simulink model "FullModel"  (R2024b)
settings: Solver=ode4  StartTime=0.0  StopTime=60  FixedStep=1e-5  RelTol=1e-3
InitFcn:
  | % Define Simulink sampling time
  | params.Tsam = 1e-5;
  | % Load frequency
  | params.f0=50;
  | %% LCL - filter design
  | % DC link voltage
  | params.Vdc=800;
  | %Switching frequency
  | params.fs=10e3;
  | params.Ts=1/params.fs;
  | params.Filter.Ls_1=1e-3;
  | params.Filter.Ls_2=0.5e-3;
  | params.Filter.Cs = 50e-6;
  | %% PI current-----------
  | params.Tresc=1e-3;
  | params.e=1;
  | params.omega=2*pi/params.Tresc;
  | params.k=1/params.Filter.Ls_1;
  | params.Kpc=2*params.e*params.omega/params.k;
  | params.Kic=params.omega^2/params.k;
  | 
  | %% PI voltage controller-----------
  | params.Tresv=10e-3;
  | params.ev=1;
  | params.omegav=2*pi/params.Tresv;
  | params.kv=1/params.Filter.Cs;
  | params.Kpv=2*params.ev*params.omegav/params.kv;
  | params.Kiv=params.omegav^2/params.kv;
  | params.Pref = 4.5e3;         % 0.5 MW
  | params.Qref = 1000;         % 0.1 Mvar
  | params.Vn   = 110;  % 22 kV line-to-line  →  phase (RMS)
  | params.wn = 2*pi*50;
  | params.Vj = 110;
  | params.XR = 1;
  | 
  | % Đặc tả cực đặt cho pole-placement
  | zeta      = 1;
  | T_setl    = 1;
  | omega_n   = 4/(zeta*T_setl);
  | p1        = -zeta*omega_n + 1i*omega_n*sqrt(1-zeta^2);
  | poles     = [p1, conj(p1), -80, -90, -100];
  | % Controller gain K
  | % K = place(A, B, p);
  | K_now = -[339.437515294446	-37.1962550049616	-155.433559437714	37.2641713114898	3289.76434330323;
  | 287.980448278270	35.5843781184771	-282.198010268474	58.4116660247888	-4058.33626972146];
  | % 3a) Conventional P-loop (fixed gains from your design)
  | Kp = 0.006383815167581;
  | Dp = 2.506338228783948e3;
  | 
  | % 3b) Conventional Q-loop (fixed gains)
  | Kq = 0.076670166944346;
  | Dq = 1.033099625954584;
undefined symbols (not defined in the file or in its folder): Filter, IP, Ls, UDP
libraries: spsSeriesRLCBranchLib x47, spsIdealSwitchLib x26, spsCurrentMeasurementLib x6, spsIGBTDiodeLib x6, rtlab x5, simulink x4, spsVoltageMeasurementLib x4, spsMeanLib x2, spsDCVoltageSourceLib x1, spsThreePhaseSourceLib x1, spsThreePhaseVIMeasurementLib x1, rtio_generic_ip x1
settings Model: Creator=Admin  LastModifiedBy=ACER
settings DataIOCC: SaveOutput=off  DSMLogging=off  SaveTime=off  ReturnWorkspaceOutputs=off
settings OptimizationCC: EfficientMapNaN2IntZero=off  AccelVerboseBuild=on
settings DebuggingCC: UnconnectedInputMsg=warning  UnconnectedOutputMsg=warning  UnconnectedLineMsg=warning
settings HardwareCC: TargetBitPerPointer=64  TargetBitPerSizeT=64  TargetBitPerPtrDiffT=64  TargetLongLongMode=on  TargetIntDivRoundTo=Zero  TargetEndianess=LittleEndian  TargetWordSize=64  TargetHWDeviceType=MATLAB Host  ProdEqTarget=off
settings ModelReferenceCC: EnableRefExpFcnMdlSchedulingChecks=on
settings SFSimCC: CustomCodeUndefinedFunction=UseInterfaceOnly
settings RTWCC: GenerateReport=on  GPUComputeCapability=3.5
settings CodeAppCC: MaxIdLength=128
settings GRTTargetCC: TargetLangStandard=C89/C90 (ANSI)  CombineOutputUpdateFcns=off  GRTInterface=on

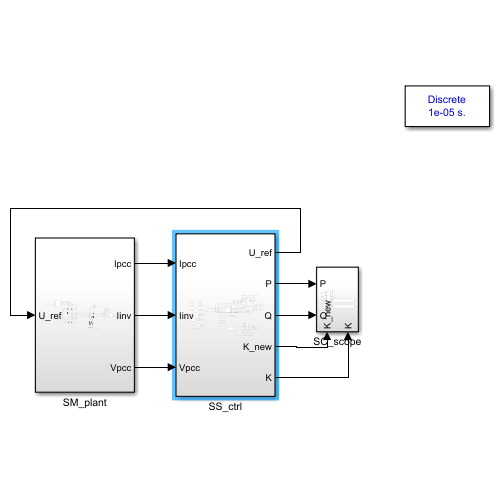
[thumbnail: Simulink's stored preview of the top-level diagram]
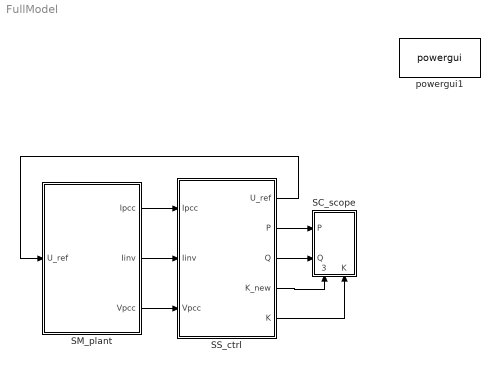
== system FullModel ==
  SC_scope : Subsystem
      settings: PortSchema="{\"entries\":[{\"content\":{\"sides\":[{\"content\":{\"connectorIds\":[\"In1\",\"In2\"]},\"type\":\"ConnectorPlacement.EquallySpacedRectSide\",\"uuid\":\"1d0fbc94-f50e-4dac-aa38-f6c6c0d58e24\"},{\"content\":{\"side\":\"RIGHT\"},\"type\":\"ConnectorPlacement.EquallySpacedRectSide\",\"uuid\":\"cb070a2d-4924-49b4-8117-60b0e85ee68e\"},{\"content\":{\"side\":\"TOP\"},\"type\":\"ConnectorPlacement.EquallySpacedRectSide\",\"uuid\":\"37bb5879-11cc-4540-93be-6819b671c3f0\"},{\"content\":{\"connectorIds\":[\"In3\",\"In4\"],\"side\":\"BOTTOM\"},\"type\":\"ConnectorPlacement.EquallySpacedRectSide\",\"uuid\":\"e4b3a2c0-2caf-4b94-9e11-126344d60f0a\"}]},\"type\":\"ConnectorPlacement.EquallySpacedConnector\",\"uuid\":\"b55f8133-fa8d-4679-9685-8775147a1bfa\"}],\"packageUris\":[\"http://schema.mathworks.com/mf0/Connector/R2020b\"],\"version\":\"1.0\"}"
  SM_plant : Subsystem
  SS_ctrl : Subsystem
  powergui1 : spspowerguiLib/powergui  Priority=1  SimulationMode=Discrete  SampleTime=1e-5  frequency=60  Iterations=50  frequencyindice=0  Pbase=100e6  ErrMax=1e-4  UnitsV=kV  UnitsW=MW  buscounter=0  FunctionMessages=off  echomessages=off  EnableUseOfTLC=off  CurrentSourceSwitches=off  DisableSnubberDevices=off  DisableRonSwitches=off  DisableVfSwitches=off  DisplayEquations=off  AutomaticDiscreteSolvers=on  SolverType=Tustin/Backward Euler (TBE)  Interpol=off  ExternalGateDelay=off  methode=off  Ts=100  x0status=blocks  SPID=on  SwTol=0  HookPort=off  NonlinearTolerance=0  nMaxIteration=15  ContinueOnMaxIteration=off  RestoreLinks=warning  ResistiveCurrentMeasurement=off  Frange=[0:2:500]  Ylog=off  Xlog=on  ShowGrid=off  save=off  variable=ZData  structure=0  ZoomFFT=off  StartTime=0.0  cycles=1  DisplayStyle=1  fundamental=60  FreqAxis=off  MaxFrequency=1000  frequencyindicesteady=1  RmsSteady=1  display=off
  wires:
  SM_plant/1(Ipcc) -> SS_ctrl/1(Ipcc)
  SM_plant/2(Iinv) -> SS_ctrl/2(Iinv)
  SM_plant/3(Vpcc) -> SS_ctrl/3(Vpcc)
  SS_ctrl/1(U_ref) -> SM_plant/1(U_ref)
  SS_ctrl/2(P) -> SC_scope/1(P)
  SS_ctrl/3(Q) -> SC_scope/2(Q)
  SS_ctrl/4(K_new) -> SC_scope/3(K_new)
  SS_ctrl/5(K) -> SC_scope/4(K)

== system FullModel/SC_scope ==
  P : Inport
  Q : Inport  Port=2
  K_new : Inport  Port=3
  K : Inport  Port=4
  Display : Display
  Display1 : Display
  OpComm : rtlab/OpComm  nbport=4  groupe_acq=1  subsys_rate=2e-4  st=0  Synchronization=on  Interpolation=on  Threshold=1.0  Missed_Data=off  Sim_Time=off  Samples=off  dynSigOut=off  from_console=0  warning_done=off  writeOpCommFile=off  Offset=off
      settings: SourceProductName=RT-LAB
  Scope : Scope  NumInputPorts=2
  wires:
  Q/1 -> OpComm/2
  P/1 -> OpComm/1
  OpComm/2 -> Scope/2
  OpComm/1 -> Scope/1
  K_new/1 -> OpComm/3
  OpComm/3 -> Display/1
  K/1 -> OpComm/4
  OpComm/4 -> Display1/1

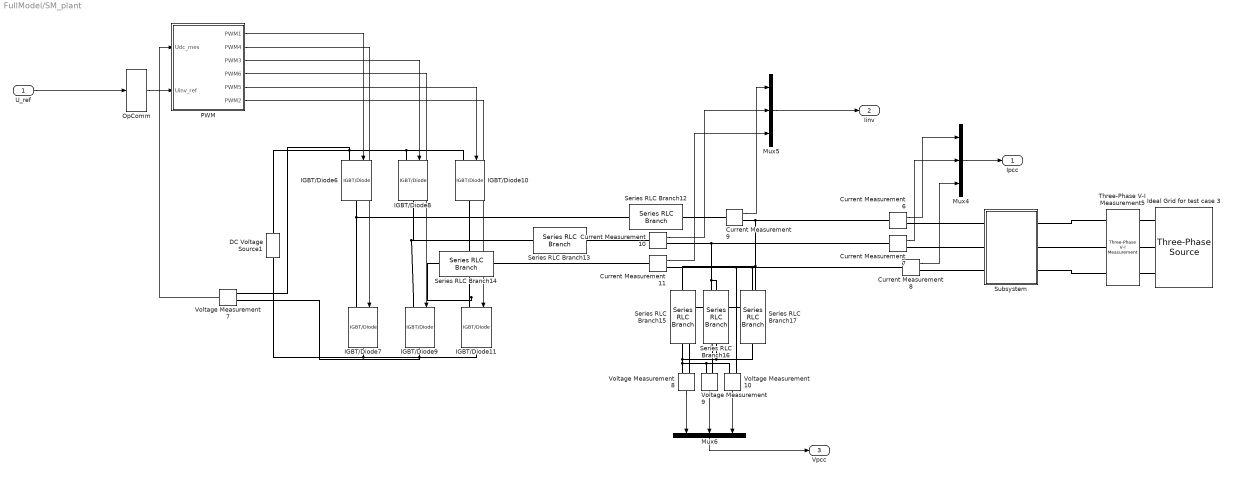
== system FullModel/SM_plant ==
  U_ref : Inport
  Current Measurement{6..11} (6 alike) : spsCurrentMeasurementLib/Current Measurement  PhasorSimulation=off  OutputType=Complex  PSBequivalent=0
  DC Voltage Source1 : spsDCVoltageSourceLib/DC Voltage Source  Amplitude=params.Vdc  Measurements=None
  IGBT/Diode{6..11} (6 alike) : spsIGBTDiodeLib/IGBT//Diode  Ron=1e-3  Rs=1e5  Cs=inf  Measurements=off
  Ideal Grid for test case 3 : spsThreePhaseSourceLib/Three-Phase Source  InternalConnection=Yg  VoltagePhases=off  Voltage=params.Vj*sqrt(3)  PhaseAngle=0  Voltage_phases=[25e3 25e3 25e3]/sqrt(3)  PhaseAngles_phases=[0 -120 +120]  Frequency=params.f0  NonIdealSource=off  SpecifyImpedance=on  Resistance=0.8929  Inductance=16.58e-3  ShortCircuitLevel=params.SCR*params.S_rated  BaseVoltage=params.Vll_rms  XRratio=params.XR  BusType=swing  Pref=1e3  Qref=0  Prefabc=[10e3, 10e3, 10e3]  Qrefabc=[0, 0, 0]  Qmin=-inf  Qmax=inf
  Mux4 : Mux  Inputs=3
  Mux5 : Mux  Inputs=3
  Mux6 : Mux  Inputs=3
  OpComm : rtlab/OpComm  nbport=1  groupe_acq=1  subsys_rate=0  st=0  Synchronization=on  Interpolation=on  Threshold=1.0  Missed_Data=off  Sim_Time=off  Samples=off  dynSigOut=off  from_console=0  warning_done=off  writeOpCommFile=off  Offset=off
      settings: SourceProductName=RT-LAB
  PWM : Subsystem
  Series RLC Branch12 : spsSeriesRLCBranchLib/Series RLC Branch  LConnTagsString=__new0  RConnTagsString=__new0  BranchType=L  Resistance=Filter.Rs_1  Inductance=params.Filter.Ls_1  SetiL0=off  InitialCurrent=1  Capacitance=1e-6  Setx0=off  InitialVoltage=0  Measurements=None
  Series RLC Branch13 : spsSeriesRLCBranchLib/Series RLC Branch  LConnTagsString=__new0  RConnTagsString=__new0  BranchType=L  Resistance=Filter.Rs_1  Inductance=params.Filter.Ls_1  SetiL0=off  InitialCurrent=1  Capacitance=1e-6  Setx0=off  InitialVoltage=0  Measurements=None
  Series RLC Branch14 : spsSeriesRLCBranchLib/Series RLC Branch  LConnTagsString=__new0  RConnTagsString=__new0  BranchType=L  Resistance=Filter.Rs_1  Inductance=params.Filter.Ls_1  SetiL0=off  InitialCurrent=1  Capacitance=1e-6  Setx0=off  InitialVoltage=0  Measurements=None
  Series RLC Branch15 : spsSeriesRLCBranchLib/Series RLC Branch  LConnTagsString=__new0  RConnTagsString=__new0  BranchType=C  Resistance=1  Inductance=Ls  SetiL0=off  InitialCurrent=0  Capacitance=params.Filter.Cs  Setx0=off  InitialVoltage=0  Measurements=None
  Series RLC Branch16 : spsSeriesRLCBranchLib/Series RLC Branch  LConnTagsString=__new0  RConnTagsString=__new0  BranchType=C  Resistance=1  Inductance=Ls  SetiL0=off  InitialCurrent=0  Capacitance=params.Filter.Cs  Setx0=off  InitialVoltage=0  Measurements=None
  Series RLC Branch17 : spsSeriesRLCBranchLib/Series RLC Branch  LConnTagsString=__new0  RConnTagsString=__new0  BranchType=C  Resistance=1  Inductance=Ls  SetiL0=off  InitialCurrent=0  Capacitance=params.Filter.Cs  Setx0=off  InitialVoltage=0  Measurements=None
  Subsystem : Subsystem
  Three-Phase V-I Measurement5 : spsThreePhaseVIMeasurementLib/Three-Phase V-I Measurement  VoltageMeasurement=no  SetLabelV=off  LabelV=Vabc  Vpu=off  VpuLL=off  CurrentMeasurement=no  SetLabelI=off  LabelI=Iabc  Ipu=off  Pbase=100e6  Vbase=500e3  OutputType=Complex  PhasorSimulation=off  PSBequivalent=0
  Voltage Measurement{7..10} (4 alike) : spsVoltageMeasurementLib/Voltage Measurement  PhasorSimulation=off  OutputType=Complex  PSBequivalent=0
  Ipcc : Outport
  Iinv : Outport  Port=2
  Vpcc : Outport  Port=3
  wires:
  Voltage Measurement8/1 -> Mux6/1
  Voltage Measurement9/1 -> Mux6/2
  Current Measurement10/1 -> Mux5/2
  Voltage Measurement10/1 -> Mux6/3
  Current Measurement6/1 -> Mux4/1
  Current Measurement7/1 -> Mux4/2
  Current Measurement8/1 -> Mux4/3
  Current Measurement11/1 -> Mux5/3
  Current Measurement9/1 -> Mux5/1
  Mux4/1 -> Ipcc/1
  Mux5/1 -> Iinv/1
  Mux6/1 -> Vpcc/1
  Voltage Measurement7/1 -> PWM/1(Udc_mes)
  U_ref/1 -> OpComm/1
  OpComm/1 -> PWM/2(Uinv_ref)
  PWM/1(PWM1) -> IGBT/Diode6/1
  PWM/3(PWM3) -> IGBT/Diode8/1
  PWM/5(PWM5) -> IGBT/Diode10/1
  PWM/2("PWM4 ") -> IGBT/Diode7/1
  PWM/4("PWM6 ") -> IGBT/Diode9/1
  PWM/6(PWM2) -> IGBT/Diode11/1
  connections:
  Three-Phase V-I Measurement5/LConn2 -- Ideal Grid for test case 3/RConn2
  Series RLC Branch13/RConn1 -- Current Measurement10/LConn1
  Series RLC Branch13/LConn1 -- IGBT/Diode9/LConn1 -- IGBT/Diode8/RConn1
  Current Measurement6/LConn1 -- Current Measurement9/RConn1 -- Voltage Measurement8/LConn1 -- Series RLC Branch15/LConn1
  Voltage Measurement10/LConn2 -- Series RLC Branch17/RConn1 -- Series RLC Branch16/RConn1 -- Series RLC Branch15/RConn1 -- Voltage Measurement8/LConn2 -- Voltage Measurement9/LConn2
  IGBT/Diode10/LConn1 -- IGBT/Diode6/LConn1 -- DC Voltage Source1/RConn1 -- Voltage Measurement7/LConn1 -- IGBT/Diode8/LConn1
  Series RLC Branch17/LConn1 -- Current Measurement8/LConn1 -- Current Measurement11/RConn1 -- Voltage Measurement10/LConn1
  Current Measurement7/LConn1 -- Voltage Measurement9/LConn1 -- Series RLC Branch16/LConn1 -- Current Measurement10/RConn1
  Current Measurement11/LConn1 -- Series RLC Branch14/RConn1
  IGBT/Diode6/RConn1 -- Series RLC Branch12/LConn1 -- IGBT/Diode7/LConn1
  Ideal Grid for test case 3/RConn1 -- Three-Phase V-I Measurement5/LConn1
  IGBT/Diode7/RConn1 -- IGBT/Diode11/RConn1 -- IGBT/Diode9/RConn1 -- Voltage Measurement7/LConn2 -- DC Voltage Source1/LConn1
  Three-Phase V-I Measurement5/LConn3 -- Ideal Grid for test case 3/RConn3
  Current Measurement9/LConn1 -- Series RLC Branch12/RConn1
  Series RLC Branch14/LConn1 -- IGBT/Diode10/RConn1 -- IGBT/Diode11/LConn1
  Subsystem/RConn1 -- Three-Phase V-I Measurement5/RConn3
  Subsystem/LConn1 -- Current Measurement6/RConn1
  Subsystem/LConn2 -- Current Measurement7/RConn1
  Subsystem/RConn2 -- Three-Phase V-I Measurement5/RConn2
  Subsystem/LConn3 -- Current Measurement8/RConn1
  Three-Phase V-I Measurement5/RConn1 -- Subsystem/RConn3

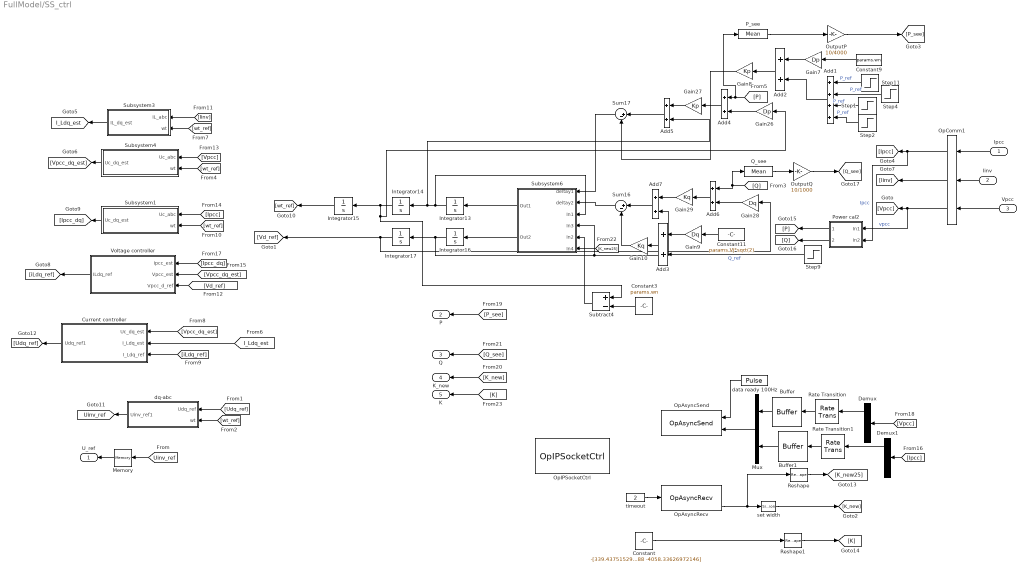
== system FullModel/SS_ctrl ==
  Ipcc : Inport
  Iinv : Inport  Port=2
  Vpcc : Inport  Port=3
  Add1 : Sum  Inputs=++++
  Add{2..7} (6 alike) : Sum
  Buffer : Buffer  N=100  OutputFrames=off
  Buffer1 : Buffer  N=100  OutputFrames=off
  Constant : Constant  Value=|
      | -[339.437515294446	-37.1962550049616	-155.433559437714	37.2641713114898	3289.76434330323
      |   287.980448278270	35.5843781184771	-282.198010268474	58.4116660247888	-4058.33626972146]
  Constant11 : Constant  Value=params.Vj*sqrt(2)
  Constant3 : Constant  Value=params.wn
  Constant9 : Constant  Value=params.wn
  Current controller : Subsystem
  Demux : Demux  Outputs=3
  Demux1 : Demux  Outputs=3
  Gain10 : Gain  Gain=Kq
  Gain26 : Gain  Gain=Dp
  Gain27 : Gain  Gain=Kp
  Gain28 : Gain  Gain=Dq
  Gain29 : Gain  Gain=Kq
  Gain7 : Gain  Gain=Dp
  Gain8 : Gain  Gain=Kp
  Gain9 : Gain  Gain=Dq
  Integrator13 : Integrator
  Integrator14 : Integrator  InitialCondition=params.wn
  Integrator15 : Integrator  InitialCondition=0.034393045493197
  Integrator16 : Integrator
  Integrator17 : Integrator  InitialCondition=110.742
  Memory : Memory
  Mux : Mux  Inputs=2
  OpAsyncRecv : rtlab/Communication/Asynchronous/OpAsyncRecv  ctl_id=1  recv_id=1  enable_param=off  fp1=1  fp2=2  fp3=3  fp4=4  fp5=5  sp1=string1  sp2=string2  sp3=string3  sp4=string4  sp5=string5  fp6=6  fp7=7
      settings: SourceProductName=RT-LAB
  OpAsyncSend : rtlab/Communication/Asynchronous/OpAsyncSend  ctl_id=1  send_id=1  mode=DONT_NEED_REPLY  enable_param=off  fp1=1  fp2=2  fp3=3  fp4=4  fp5=5  sp1=string1  sp2=string2  sp3=string3  sp4=string4  sp5=string5
      settings: SourceProductName=RT-LAB
  OpComm1 : rtlab/OpComm  nbport=3  groupe_acq=1  subsys_rate=0  st=0  Synchronization=on  Interpolation=on  Threshold=1.0  Missed_Data=off  Sim_Time=off  Samples=off  dynSigOut=off  from_console=0  warning_done=off  writeOpCommFile=off  Offset=off
      settings: SourceProductName=RT-LAB
  OpIPSocketCtrl : rtio_generic_ip/OpIPSocketCtrl  ctl_id=1  proto=UDP/IP  ip_addr_remote=192.168.5.15  ip_port_remote=5556  ip_port_local=6000  ip_addr_mcast=0.0.0.0  exe_name=AsyncIP
      settings: SourceProductName=IP
  OutputP : Gain  Gain=10/4000
  OutputQ : Gain  Gain=10/1000
  P_see : spsMeanLib/Mean  Freq=60  Vinit=0  Ts=0
  Power cal2 : Subsystem
  Q_see : spsMeanLib/Mean  Freq=60  Vinit=0  Ts=0
  Rate Transition : RateTransition  OutPortSampleTime=2e-4
  Rate Transition1 : RateTransition  OutPortSampleTime=2e-4
  Reshape : Reshape  OutputDimensionality=Customize  OutputDimensions=[2,5]
  Reshape1 : Reshape  OutputDimensions=[1 10]
  Step1 : Step  Time=90  After=0.5e3  SampleTime=0
  Step11 : Step  Time=30  Before=3e3  After=3.5e3  SampleTime=0
  Step2 : Step  Time=110  After=0.5e3  SampleTime=0
  Step4 : Step  Time=50  After=0  SampleTime=0
  Step9 : Step  Time=70  Before=1e3  After=1.5e3  SampleTime=0
  Subsystem1 : Subsystem
  Subsystem3 : Subsystem
  Subsystem4 : Subsystem
  Subsystem6 : Subsystem
  Subtract4 : Sum  Inputs=+-
  Sum16 : Sum  Inputs=|+-
  Sum17 : Sum  Inputs=|+-
  Voltage controller : Subsystem
  data ready 100Hz : DiscretePulseGenerator  Period=2500  PulseWidth=101  SampleTime=2e-4
  dq-abc : Subsystem
  set width : SignalSpecification  Dimensions=10
  timeout : Constant  Value=2
  U_ref : Outport
  P : Outport  Port=2
  Q : Outport  Port=3
  K_new : Outport  Port=4
  K : Outport  Port=5
  tag scope: I_Ldq_est=global, Uinv_ref=global
  wires:
  Sum17/1 -> Subsystem6/1(deltay1)
  Add7/1 -> Sum16/1
  Gain29/1 -> Add7/1
  Add4/1 -> Gain27/1
  Integrator17/1 -> [Vd_ref], Gain28/1
  [P] -> P_see/1, Add4/1
  Add2/1 -> Gain8/1
  Gain10/1 -> Sum16/2
  Subsystem6/2(Out2) -> Integrator16/1
  Gain9/1 -> Add3/1
  [Q] -> Add6/1, Q_see/1
  Gain8/1 -> Sum17/2
  Constant3/1 -> Subtract4/2
  Add6/1 -> Gain29/1
  Gain28/1 -> Add6/2
  Add3/1 -> Gain10/1
  Gain27/1 -> Add5/1
  Constant11/1 -> Gain9/1
  Integrator15/1 -> [wt_ref]
  Integrator16/1 -> Subsystem6/4(In3), Add7/2, Integrator17/1
  Subsystem6/1(Out1) -> Integrator13/1
  Add5/1 -> Sum17/1
  OpComm1/3 -> [Vpcc], Power cal2/1(In1)  "vpcc"
  Integrator13/1 -> Integrator14/1, Add5/2, Subsystem6/3(In1)
  Integrator14/1 -> Subtract4/1, Gain26/1, Integrator15/1
  Gain7/1 -> Add2/1
  Gain26/1 -> Add4/2
  Power cal2/1(deltay1) -> [P]
  Constant9/1 -> Gain7/1
  Subtract4/1 -> Subsystem6/5(In2)
  Sum16/1 -> Subsystem6/2(deltay2)
  Power cal2/2(deltay2) -> [Q]
  [Vd_ref] -> Voltage controller/3(Vpcc_d_ref)
  [Ipcc] -> Subsystem1/1(Uc_abc)
  [Vpcc] -> Subsystem4/1(Uc_abc)
  Subsystem1/1(Uc_dq_est) -> [Ipcc_dq]
  [wt_ref] -> Subsystem1/2(wt)
  [iLdq_ref] -> Current controller/3(I_Ldq_ref)
  [Vpcc_dq_est] -> Voltage controller/2(Vpcc_est)
  Voltage controller/1(ILdq_ref) -> [iLdq_ref]
  [Ipcc_dq] -> Voltage controller/1(Ipcc_est)
  [Udq_ref] -> dq-abc/1(Udq_ref)
  [wt_ref] -> Subsystem4/2(wt)
  Subsystem3/1(IL_dq_est) -> [I_Ldq_est]
  [Iinv] -> Subsystem3/1(IL_abc)
  [wt_ref] -> dq-abc/2(wt)
  dq-abc/1(Uinv_ref1) -> [Uinv_ref]
  [wt_ref] -> Subsystem3/2(wt)
  Current controller/1(Udq_ref1) -> [Udq_ref]
  Subsystem4/1(Uc_dq_est) -> [Vpcc_dq_est]
  [I_Ldq_est] -> Current controller/2(I_Ldq_est)
  [Vpcc_dq_est] -> Current controller/1(Uc_dq_est)
  Vpcc/1 -> OpComm1/3
  Q_see/1 -> OutputQ/1
  [P_see] -> P/1
  [Q_see] -> Q/1
  Step9/1 -> Add3/2  "Q_ref"
  [Uinv_ref] -> Memory/1
  Ipcc/1 -> OpComm1/1
  Iinv/1 -> OpComm1/2
  OpComm1/1 -> Power cal2/2(In2), [Ipcc]  "Ipcc"
  Memory/1 -> U_ref/1
  [K_new] -> K_new/1
  OpComm1/2 -> [Iinv]
  Rate Transition/1 -> Buffer/1
  Rate Transition1/1 -> Buffer1/1
  [Vpcc] -> Demux/1
  [Ipcc] -> Demux1/1
  Demux1/1 -> Rate Transition1/1
  Demux/1 -> Rate Transition/1
  Buffer/1 -> Mux/1
  Buffer1/1 -> Mux/2
  Mux/1 -> OpAsyncSend/2
  data ready 100Hz/1 -> OpAsyncSend/1
  timeout/1 -> OpAsyncRecv/1
  set width/1 -> [K_new]
  [K_new25] -> Subsystem6/6(In4)
  Reshape/1 -> [K_new25]
  OpAsyncRecv/3 -> Reshape/1, set width/1
  Constant/1 -> Reshape1/1
  Reshape1/1 -> [K]
  [K] -> K/1
  P_see/1 -> OutputP/1
  OutputQ/1 -> [Q_see]
  OutputP/1 -> [P_see]
  Step11/1 -> Add1/1  "P_ref"
  Step4/1 -> Add1/2  "P_ref"
  Add1/1 -> Add2/2
  Step2/1 -> Add1/4  "P_ref"
  Step1/1 -> Add1/3  "P_ref"

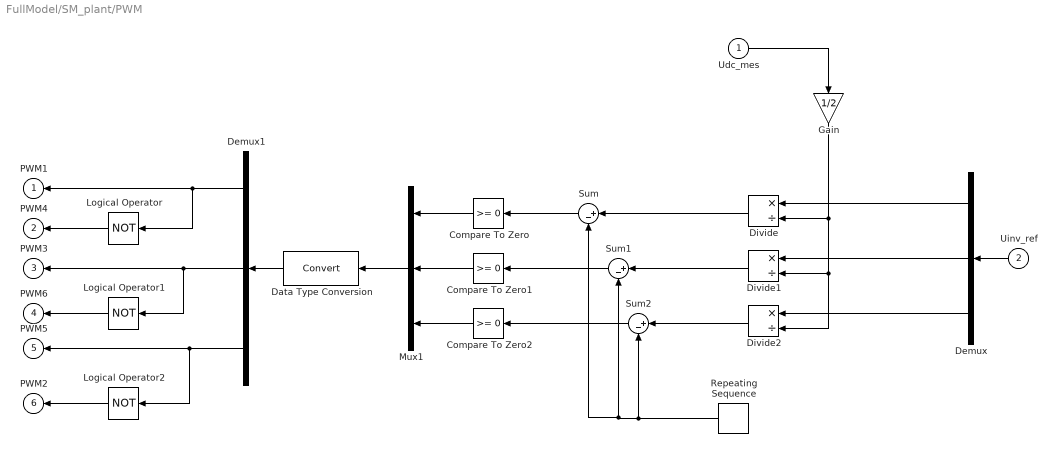
== system FullModel/SM_plant/PWM ==
  Udc_mes : Inport
  Uinv_ref : Inport  Port=2
  Compare To Zero : simulink/Logic and Bit Operations/Compare To Zero  relop=>=  OutDataTypeStr=boolean
  Compare To Zero1 : simulink/Logic and Bit Operations/Compare To Zero  relop=>=  OutDataTypeStr=boolean
  Compare To Zero2 : simulink/Logic and Bit Operations/Compare To Zero  relop=>=  OutDataTypeStr=boolean
  Data Type Conversion : DataTypeConversion  SaturateOnIntegerOverflow=off  RndMeth=Floor
  Demux : Demux  Outputs=3
  Demux1 : Demux  Outputs=3
  Divide : Product  Inputs=*/
  Divide1 : Product  Inputs=*/
  Divide2 : Product  Inputs=*/
  Gain : Gain  Gain=1/2
  Logical Operator : Logic  Operator=NOT  AllPortsSameDT=off  OutDataTypeStr=boolean
  Logical Operator1 : Logic  Operator=NOT  AllPortsSameDT=off  OutDataTypeStr=boolean
  Logical Operator2 : Logic  Operator=NOT  AllPortsSameDT=off  OutDataTypeStr=boolean
  Mux1 : Mux  Inputs=3
  Repeating Sequence : simulink/Sources/Repeating Sequence  rep_seq_t=[0 params.Ts/2 params.Ts]  rep_seq_y=[-1 1 -1]
  Sum : Sum  Inputs=|+-
  Sum1 : Sum  Inputs=|+-
  Sum2 : Sum  Inputs=|+-
  PWM1 : Outport  InitialOutput=0  VectorParamsAs1DForOutWhenUnconnected=off
  "PWM4 " : Outport  Port=2  InitialOutput=0  VectorParamsAs1DForOutWhenUnconnected=off
  PWM3 : Outport  Port=3  InitialOutput=0  VectorParamsAs1DForOutWhenUnconnected=off
  "PWM6 " : Outport  Port=4  InitialOutput=0  VectorParamsAs1DForOutWhenUnconnected=off
  PWM5 : Outport  Port=5  InitialOutput=0  VectorParamsAs1DForOutWhenUnconnected=off
  PWM2 : Outport  Port=6  InitialOutput=0  VectorParamsAs1DForOutWhenUnconnected=off
  wires:
  Repeating Sequence/1 -> Sum/2, Sum1/2, Sum2/2
  Sum1/1 -> Compare To Zero1/1
  Mux1/1 -> Data Type Conversion/1
  Divide2/1 -> Sum2/1
  Divide/1 -> Sum/1
  Logical Operator/1 -> "PWM4 "/1
  Sum2/1 -> Compare To Zero2/1
  Divide1/1 -> Sum1/1
  Demux/1 -> Divide/1
  Uinv_ref/1 -> Demux/1
  Demux1/2 -> PWM3/1, Logical Operator1/1
  Demux1/3 -> PWM5/1, Logical Operator2/1
  Compare To Zero2/1 -> Mux1/3
  Compare To Zero1/1 -> Mux1/2
  Demux/2 -> Divide1/1
  Logical Operator2/1 -> PWM2/1
  Logical Operator1/1 -> "PWM6 "/1
  Udc_mes/1 -> Gain/1
  Demux/3 -> Divide2/1
  Sum/1 -> Compare To Zero/1
  Gain/1 -> Divide/2, Divide1/2, Divide2/2
  Demux1/1 -> PWM1/1, Logical Operator/1
  Data Type Conversion/1 -> Demux1/1
  Compare To Zero/1 -> Mux1/1

== system FullModel/SM_plant/Subsystem ==
  Clock1 : Clock
      settings: Decimation=200
  MATLAB Function2 : MATLAB Function  TreatAsAtomicUnit=on
  Subsystem : Subsystem
  Subsystem1 : Subsystem  Commented=on
  Subsystem2 : Subsystem  Commented=on
  Subsystem3 : Subsystem
  Subsystem4 : Subsystem
  "C     " : PMIOPort  Side=Right
  A : PMIOPort  Port=2  Side=Left
  B : PMIOPort  Port=3  Side=Left
  "B  " : PMIOPort  Port=4  Side=Right
  "  C " : PMIOPort  Port=5  Side=Left
  "A     " : PMIOPort  Port=6  Side=Right
  wires:
  Clock1/1 -> MATLAB Function2/1(t)
  MATLAB Function2/1(s) -> Subsystem4/1(In1), Subsystem3/1(In1), Subsystem/1(In1)
  connections:
  Subsystem3/LConn1 -- B/RConn1
  Subsystem3/RConn1 -- "B  "/RConn1
  Subsystem4/RConn1 -- "A     "/RConn1
  Subsystem4/LConn1 -- A/RConn1
  Subsystem/LConn1 -- "  C "/RConn1
  Subsystem/RConn1 -- "C     "/RConn1

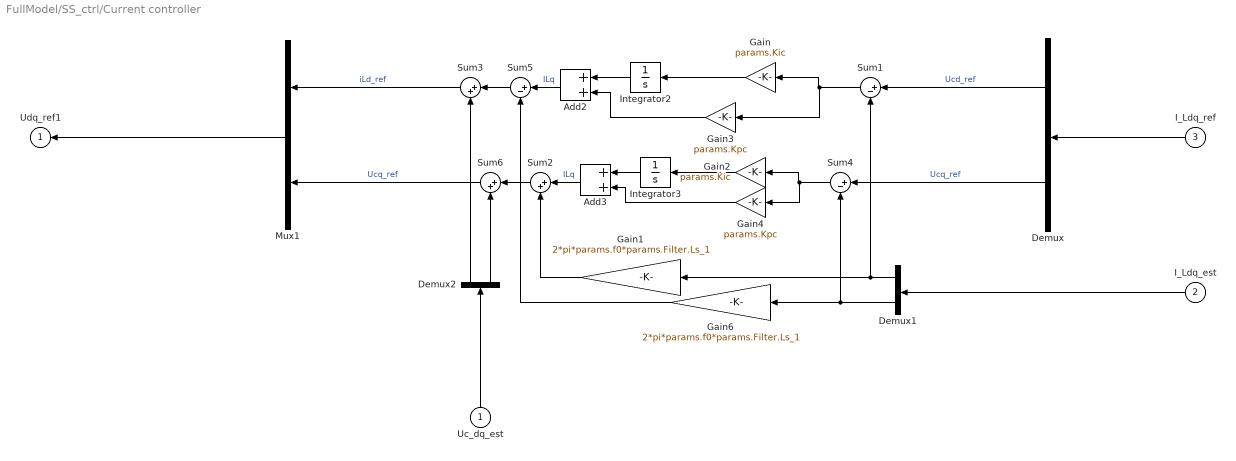
== system FullModel/SS_ctrl/Current controller ==
  Uc_dq_est : Inport
  I_Ldq_est : Inport  Port=2
  I_Ldq_ref : Inport  Port=3
  Add2 : Sum
  Add3 : Sum
  Demux : Demux  Outputs=2
  Demux1 : Demux  Outputs=2
  Demux2 : Demux  Outputs=2
  Gain : Gain  Gain=params.Kic
  Gain1 : Gain  Gain=2*pi*params.f0*params.Filter.Ls_1
  Gain2 : Gain  Gain=params.Kic
  Gain3 : Gain  Gain=params.Kpc
  Gain4 : Gain  Gain=params.Kpc
  Gain6 : Gain  Gain=2*pi*params.f0*params.Filter.Ls_1
  Integrator2 : Integrator
  Integrator3 : Integrator
  Mux1 : Mux  Inputs=2
  Sum1 : Sum  Inputs=|+-
  Sum2 : Sum  Inputs=|++
  Sum3 : Sum  Inputs=|++
  Sum4 : Sum  Inputs=|+-
  Sum5 : Sum  Inputs=|+-
  Sum6 : Sum  Inputs=|++
  Udq_ref1 : Outport  InitialOutput=0  VectorParamsAs1DForOutWhenUnconnected=off
  wires:
  I_Ldq_ref/1 -> Demux/1
  Demux2/2 -> Sum6/2
  Sum2/1 -> Sum6/1
  I_Ldq_est/1 -> Demux1/1
  Sum3/1 -> Mux1/1  "iLd_ref"
  Demux/2 -> Sum4/1  "Ucq_ref"
  Gain1/1 -> Sum2/2
  Sum6/1 -> Mux1/2  "Ucq_ref"
  Demux2/1 -> Sum3/2
  Sum5/1 -> Sum3/1
  Mux1/1 -> Udq_ref1/1
  Gain6/1 -> Sum5/2
  Uc_dq_est/1 -> Demux2/1
  Demux1/2 -> Gain6/1, Sum4/2
  Demux/1 -> Sum1/1  "Ucd_ref"
  Demux1/1 -> Sum1/2, Gain1/1
  Add2/1 -> Sum5/1  "ILq"
  Add3/1 -> Sum2/1  "ILq"
  Integrator2/1 -> Add2/1
  Integrator3/1 -> Add3/1
  Gain/1 -> Integrator2/1
  Sum1/1 -> Gain3/1, Gain/1
  Gain2/1 -> Integrator3/1
  Sum4/1 -> Gain4/1, Gain2/1
  Gain3/1 -> Add2/2
  Gain4/1 -> Add3/2

== system FullModel/SS_ctrl/Power cal2 ==
  In1 : Inport
  In2 : Inport  Port=2
  Demux10 : Demux  Outputs=3
  Demux11 : Demux  Outputs=3
  Subsystem8 : Subsystem
  Subsystem9 : Subsystem
  p3 : Subsystem
  q3 : Subsystem
  deltay1 : Outport
  deltay2 : Outport  Port=2
  wires:
  In1/1 -> Demux11/1
  In2/1 -> Demux10/1
  q3/1(deltay2) -> deltay2/1
  Demux10/1 -> Subsystem8/1(xa)
  Demux11/2 -> Subsystem9/2(xb)
  Demux11/1 -> Subsystem9/1(xa)
  Subsystem9/2(xbeta) -> q3/2(Beta), p3/2(Beta)
  p3/1(deltay1) -> deltay1/1
  Demux10/3 -> Subsystem8/3(xc)
  Subsystem9/1(xalpha) -> q3/1(Alpha), p3/1(Alpha)
  Demux10/2 -> Subsystem8/2(xb)
  Subsystem8/2(xbeta) -> q3/4(xbeta), p3/4(xbeta)
  Demux11/3 -> Subsystem9/3(xc)
  Subsystem8/1(xalpha) -> q3/3(xalpha), p3/3(xalpha)

== system FullModel/SS_ctrl/Subsystem1 ==
  Uc_abc : Inport
  wt : Inport  Port=2
  Demux : Demux  Outputs=3
  Mux1 : Mux  Inputs=2
  Subsystem1 : Subsystem
  Subsystem2 : Subsystem
  Uc_dq_est : Outport  InitialOutput=0  VectorParamsAs1DForOutWhenUnconnected=off
  wires:
  Mux1/1 -> Uc_dq_est/1
  wt/1 -> Subsystem2/3(wt)
  Demux/3 -> Subsystem1/3(xc)
  Subsystem2/1(xd) -> Mux1/1
  Subsystem1/2(xbeta) -> Subsystem2/2(xbeta)
  Demux/1 -> Subsystem1/1(xa)
  Uc_abc/1 -> Demux/1
  Subsystem1/1(xalpha) -> Subsystem2/1(xalpha)
  Demux/2 -> Subsystem1/2(xb)
  Subsystem2/2(xq) -> Mux1/2

== system FullModel/SS_ctrl/Subsystem3 ==
  IL_abc : Inport
  wt : Inport  Port=2
  Demux : Demux  Outputs=3
  Mux1 : Mux  Inputs=2
  Subsystem1 : Subsystem
  Subsystem2 : Subsystem
  IL_dq_est : Outport  InitialOutput=0  VectorParamsAs1DForOutWhenUnconnected=off
  wires:
  Demux/3 -> Subsystem1/3(xc)
  IL_abc/1 -> Demux/1
  wt/1 -> Subsystem2/3(wt)
  Demux/1 -> Subsystem1/1(xa)
  Subsystem1/2(xbeta) -> Subsystem2/2(xbeta)
  Mux1/1 -> IL_dq_est/1
  Demux/2 -> Subsystem1/2(xb)
  Subsystem1/1(xalpha) -> Subsystem2/1(xalpha)
  Subsystem2/2(xq) -> Mux1/2
  Subsystem2/1(xd) -> Mux1/1

== system FullModel/SS_ctrl/Subsystem4 ==
  Uc_abc : Inport
  wt : Inport  Port=2
  Demux : Demux  Outputs=3
  Mux1 : Mux  Inputs=2
  Subsystem1 : Subsystem
  Subsystem2 : Subsystem
  Uc_dq_est : Outport  InitialOutput=0  VectorParamsAs1DForOutWhenUnconnected=off
  wires:
  Subsystem2/2(xq) -> Mux1/2
  Demux/2 -> Subsystem1/2(xb)
  Subsystem1/1(xalpha) -> Subsystem2/1(xalpha)
  Uc_abc/1 -> Demux/1
  Demux/1 -> Subsystem1/1(xa)
  Subsystem1/2(xbeta) -> Subsystem2/2(xbeta)
  Subsystem2/1(xd) -> Mux1/1
  Demux/3 -> Subsystem1/3(xc)
  wt/1 -> Subsystem2/3(wt)
  Mux1/1 -> Uc_dq_est/1

== system FullModel/SS_ctrl/Subsystem6 ==
  deltay1 : Inport
  deltay2 : Inport  Port=2
  In1 : Inport  Port=3
  In3 : Inport  Port=4
  In2 : Inport  Port=5
  In4 : Inport  Port=6
  Demux10 : Demux  Outputs=2
  Mux7 : Mux  Inputs=5
  Product : Product  Multiplication=Matrix(*)
  Out1 : Outport
  Out2 : Outport  Port=2
  wires:
  Product/1 -> Demux10/1
  In2/1 -> Mux7/5
  In3/1 -> Mux7/4
  Mux7/1 -> Product/2
  Demux10/2 -> Out2/1
  deltay1/1 -> Mux7/1
  deltay2/1 -> Mux7/2
  In1/1 -> Mux7/3
  Demux10/1 -> Out1/1
  In4/1 -> Product/1

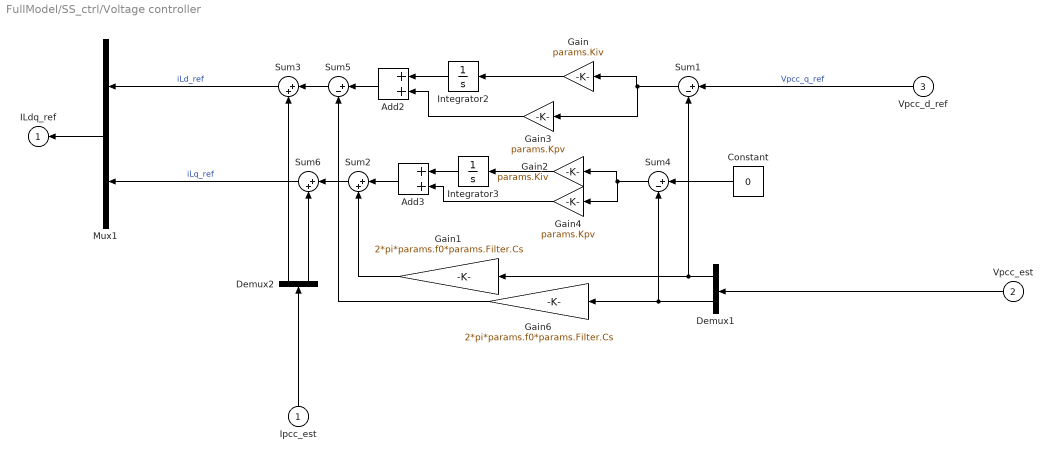
== system FullModel/SS_ctrl/Voltage controller ==
  Ipcc_est : Inport
  Vpcc_est : Inport  Port=2
  Vpcc_d_ref : Inport  Port=3
  Add2 : Sum
  Add3 : Sum
  Constant : Constant  Value=0
  Demux1 : Demux  Outputs=2
  Demux2 : Demux  Outputs=2
  Gain : Gain  Gain=params.Kiv
  Gain1 : Gain  Gain=2*pi*params.f0*params.Filter.Cs
  Gain2 : Gain  Gain=params.Kiv
  Gain3 : Gain  Gain=params.Kpv
  Gain4 : Gain  Gain=params.Kpv
  Gain6 : Gain  Gain=2*pi*params.f0*params.Filter.Cs
  Integrator2 : Integrator
  Integrator3 : Integrator
  Mux1 : Mux  Inputs=2
  Sum1 : Sum  Inputs=|+-
  Sum2 : Sum  Inputs=|++
  Sum3 : Sum  Inputs=|++
  Sum4 : Sum  Inputs=|+-
  Sum5 : Sum  Inputs=|+-
  Sum6 : Sum  Inputs=|++
  ILdq_ref : Outport  InitialOutput=0  VectorParamsAs1DForOutWhenUnconnected=off
  wires:
  Gain4/1 -> Add3/2
  Gain3/1 -> Add2/2
  Sum4/1 -> Gain2/1, Gain4/1
  Gain2/1 -> Integrator3/1
  Sum1/1 -> Gain/1, Gain3/1
  Gain/1 -> Integrator2/1
  Integrator3/1 -> Add3/1
  Integrator2/1 -> Add2/1
  Add3/1 -> Sum2/1
  Add2/1 -> Sum5/1
  Demux1/1 -> Gain1/1, Sum1/2
  Demux1/2 -> Sum4/2, Gain6/1
  Ipcc_est/1 -> Demux2/1
  Gain6/1 -> Sum5/2
  Mux1/1 -> ILdq_ref/1
  Sum5/1 -> Sum3/1
  Demux2/1 -> Sum3/2
  Sum6/1 -> Mux1/2  "iLq_ref"
  Gain1/1 -> Sum2/2
  Sum3/1 -> Mux1/1  "iLd_ref"
  Vpcc_est/1 -> Demux1/1
  Sum2/1 -> Sum6/1
  Demux2/2 -> Sum6/2
  Vpcc_d_ref/1 -> Sum1/1  "Vpcc_q_ref"
  Constant/1 -> Sum4/1

== system FullModel/SS_ctrl/dq-abc ==
  Udq_ref : Inport
  wt : Inport  Port=2
  Subsystem2 : Subsystem
  Subsystem3 : Subsystem
  Uinv_ref1 : Outport  InitialOutput=0  VectorParamsAs1DForOutWhenUnconnected=off
  wires:
  wt/1 -> Subsystem2/2(wt)
  Subsystem2/1(xalbe) -> Subsystem3/1(xalbe)
  Subsystem3/1(xabc) -> Uinv_ref1/1
  Udq_ref/1 -> Subsystem2/1(xdq)

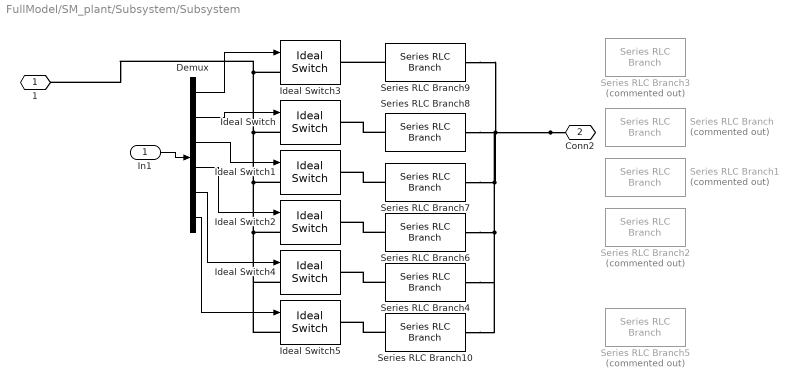
== system FullModel/SM_plant/Subsystem/Subsystem ==
  In1 : Inport
  Demux : Demux  Outputs=6
  Ideal Switch{,1..5} (6 alike) : spsIdealSwitchLib/Ideal Switch  Ron=0.001  Lon=0  IC=0  Rs=1e5  Cs=inf  Measurements=off
  Series RLC Branch : spsSeriesRLCBranchLib/Series RLC Branch  Commented=on  LConnTagsString=__new0  RConnTagsString=__new0  BranchType=RL  Resistance=0.241464008201299  Inductance=0.0115290571452056  SetiL0=off  InitialCurrent=0  Capacitance=1e-6  Setx0=off  InitialVoltage=0  Measurements=None
  Series RLC Branch1 : spsSeriesRLCBranchLib/Series RLC Branch  Commented=on  LConnTagsString=__new0  RConnTagsString=__new0  BranchType=RL  Resistance=0.0603660020503248  Inductance=0.00288226428630141  SetiL0=off  InitialCurrent=0  Capacitance=1e-6  Setx0=off  InitialVoltage=0  Measurements=None
  Series RLC Branch{4,6..10} (6 alike) : spsSeriesRLCBranchLib/Series RLC Branch  LConnTagsString=__new0  RConnTagsString=__new0  BranchType=RL  Resistance=1.28339880785358  Inductance=0.00408518528456287  SetiL0=off  InitialCurrent=0  Capacitance=1e-6  Setx0=off  InitialVoltage=0  Measurements=None
  Series RLC Branch2 : spsSeriesRLCBranchLib/Series RLC Branch  Commented=on  LConnTagsString=__new0  RConnTagsString=__new0  BranchType=RL  Resistance=0.0402440013668832  Inductance=0.00192150952420094  SetiL0=off  InitialCurrent=0  Capacitance=1e-6  Setx0=off  InitialVoltage=0  Measurements=None
  Series RLC Branch3 : spsSeriesRLCBranchLib/Series RLC Branch  Commented=on  LConnTagsString=__new0  RConnTagsString=__new0  BranchType=RL  Resistance=0.241464008201299  Inductance=0.0115290571452056  SetiL0=off  InitialCurrent=0  Capacitance=1e-6  Setx0=off  InitialVoltage=0  Measurements=None
  Series RLC Branch5 : spsSeriesRLCBranchLib/Series RLC Branch  Commented=on  LConnTagsString=__new0  RConnTagsString=__new0  BranchType=RL  Resistance=0.120732004100650  Inductance=0.00576452857260281  SetiL0=off  InitialCurrent=0  Capacitance=1e-6  Setx0=off  InitialVoltage=0  Measurements=None
  1 : PMIOPort  Side=Left
  Conn2 : PMIOPort  Port=2  Side=Right
  wires:
  In1/1 -> Demux/1
  Demux/4 -> Ideal Switch2/1
  Demux/3 -> Ideal Switch1/1
  Demux/2 -> Ideal Switch/1
  Demux/1 -> Ideal Switch3/1
  Demux/5 -> Ideal Switch4/1
  Demux/6 -> Ideal Switch5/1
  connections:
  Ideal Switch/LConn1 -- Ideal Switch3/LConn1 -- 1/RConn1 -- Ideal Switch5/LConn1 -- Ideal Switch4/LConn1 -- Ideal Switch2/LConn1 -- Ideal Switch1/LConn1
  Conn2/RConn1 -- Series RLC Branch9/RConn1 -- Series RLC Branch8/RConn1 -- Series RLC Branch7/RConn1 -- Series RLC Branch6/RConn1 -- Series RLC Branch10/RConn1 -- Series RLC Branch4/RConn1
  Series RLC Branch7/LConn1 -- Ideal Switch1/RConn1
  Series RLC Branch8/LConn1 -- Ideal Switch/RConn1
  Series RLC Branch6/LConn1 -- Ideal Switch2/RConn1
  Series RLC Branch9/LConn1 -- Ideal Switch3/RConn1
  Series RLC Branch4/LConn1 -- Ideal Switch4/RConn1
  Series RLC Branch10/LConn1 -- Ideal Switch5/RConn1

== system FullModel/SM_plant/Subsystem/Subsystem1 ==
  In1 : Inport
  Demux : Demux
  Ideal Switch{,1..3} (4 alike) : spsIdealSwitchLib/Ideal Switch  Ron=0.001  Lon=0  IC=0  Rs=1e5  Cs=inf  Measurements=off
  Series RLC Branch : spsSeriesRLCBranchLib/Series RLC Branch  LConnTagsString=__new0  RConnTagsString=__new0  BranchType=RL  Resistance=0.241464008201299  Inductance=0.0115290571452056  SetiL0=off  InitialCurrent=0  Capacitance=1e-6  Setx0=off  InitialVoltage=0  Measurements=None
  Series RLC Branch1 : spsSeriesRLCBranchLib/Series RLC Branch  LConnTagsString=__new0  RConnTagsString=__new0  BranchType=RL  Resistance=0.0603660020503248  Inductance=0.00288226428630141  SetiL0=off  InitialCurrent=0  Capacitance=1e-6  Setx0=off  InitialVoltage=0  Measurements=None
  Series RLC Branch2 : spsSeriesRLCBranchLib/Series RLC Branch  LConnTagsString=__new0  RConnTagsString=__new0  BranchType=RL  Resistance=0.0402440013668832  Inductance=0.00192150952420094  SetiL0=off  InitialCurrent=0  Capacitance=1e-6  Setx0=off  InitialVoltage=0  Measurements=None
  Series RLC Branch3 : spsSeriesRLCBranchLib/Series RLC Branch  LConnTagsString=__new0  RConnTagsString=__new0  BranchType=RL  Resistance=0.241464008201299  Inductance=0.0115290571452056  SetiL0=off  InitialCurrent=0  Capacitance=1e-6  Setx0=off  InitialVoltage=0  Measurements=None
  1 : PMIOPort  Side=Left
  Conn2 : PMIOPort  Port=2  Side=Right
  wires:
  Demux/1 -> Ideal Switch3/1
  Demux/2 -> Ideal Switch/1
  Demux/3 -> Ideal Switch1/1
  Demux/4 -> Ideal Switch2/1
  In1/1 -> Demux/1
  connections:
  Series RLC Branch3/LConn1 -- Ideal Switch3/RConn1
  Series RLC Branch2/LConn1 -- Ideal Switch2/RConn1
  Series RLC Branch/LConn1 -- Ideal Switch/RConn1
  Series RLC Branch1/LConn1 -- Ideal Switch1/RConn1
  Series RLC Branch3/RConn1 -- Series RLC Branch1/RConn1 -- Series RLC Branch2/RConn1 -- Conn2/RConn1 -- Series RLC Branch/RConn1
  Ideal Switch3/LConn1 -- Ideal Switch1/LConn1 -- Ideal Switch2/LConn1 -- Ideal Switch/LConn1 -- 1/RConn1

== system FullModel/SM_plant/Subsystem/Subsystem2 ==
  In1 : Inport
  Demux : Demux
  Ideal Switch{,1..3} (4 alike) : spsIdealSwitchLib/Ideal Switch  Ron=0.001  Lon=0  IC=0  Rs=1e5  Cs=inf  Measurements=off
  Series RLC Branch : spsSeriesRLCBranchLib/Series RLC Branch  LConnTagsString=__new0  RConnTagsString=__new0  BranchType=RL  Resistance=0.241464008201299  Inductance=0.0115290571452056  SetiL0=off  InitialCurrent=0  Capacitance=1e-6  Setx0=off  InitialVoltage=0  Measurements=None
  Series RLC Branch1 : spsSeriesRLCBranchLib/Series RLC Branch  LConnTagsString=__new0  RConnTagsString=__new0  BranchType=RL  Resistance=0.0603660020503248  Inductance=0.00288226428630141  SetiL0=off  InitialCurrent=0  Capacitance=1e-6  Setx0=off  InitialVoltage=0  Measurements=None
  Series RLC Branch2 : spsSeriesRLCBranchLib/Series RLC Branch  LConnTagsString=__new0  RConnTagsString=__new0  BranchType=RL  Resistance=0.0402440013668832  Inductance=0.00192150952420094  SetiL0=off  InitialCurrent=0  Capacitance=1e-6  Setx0=off  InitialVoltage=0  Measurements=None
  Series RLC Branch3 : spsSeriesRLCBranchLib/Series RLC Branch  LConnTagsString=__new0  RConnTagsString=__new0  BranchType=RL  Resistance=0.241464008201299  Inductance=0.0115290571452056  SetiL0=off  InitialCurrent=0  Capacitance=1e-6  Setx0=off  InitialVoltage=0  Measurements=None
  1 : PMIOPort  Side=Left
  Conn2 : PMIOPort  Port=2  Side=Right
  wires:
  In1/1 -> Demux/1
  Demux/4 -> Ideal Switch2/1
  Demux/3 -> Ideal Switch1/1
  Demux/2 -> Ideal Switch/1
  Demux/1 -> Ideal Switch3/1
  connections:
  1/RConn1 -- Ideal Switch/LConn1 -- Ideal Switch2/LConn1 -- Ideal Switch1/LConn1 -- Ideal Switch3/LConn1
  Series RLC Branch/RConn1 -- Conn2/RConn1 -- Series RLC Branch2/RConn1 -- Series RLC Branch1/RConn1 -- Series RLC Branch3/RConn1
  Series RLC Branch1/LConn1 -- Ideal Switch1/RConn1
  Series RLC Branch/LConn1 -- Ideal Switch/RConn1
  Series RLC Branch2/LConn1 -- Ideal Switch2/RConn1
  Series RLC Branch3/LConn1 -- Ideal Switch3/RConn1

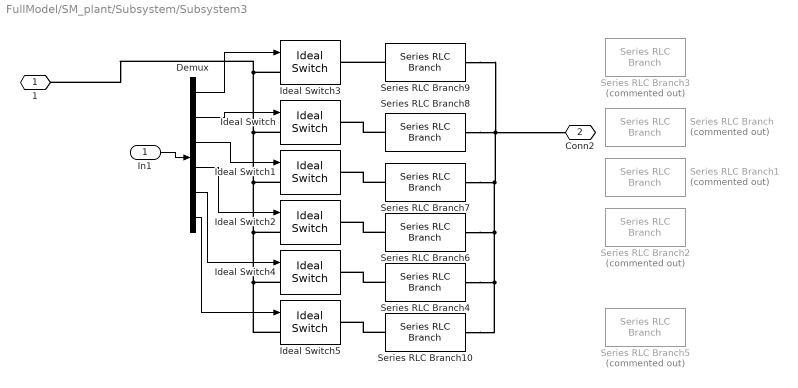
== system FullModel/SM_plant/Subsystem/Subsystem3 ==
  In1 : Inport
  Demux : Demux  Outputs=6
  Ideal Switch{,1..5} (6 alike) : spsIdealSwitchLib/Ideal Switch  Ron=0.001  Lon=0  IC=0  Rs=1e5  Cs=inf  Measurements=off
  Series RLC Branch : spsSeriesRLCBranchLib/Series RLC Branch  Commented=on  LConnTagsString=__new0  RConnTagsString=__new0  BranchType=RL  Resistance=0.241464008201299  Inductance=0.0115290571452056  SetiL0=off  InitialCurrent=0  Capacitance=1e-6  Setx0=off  InitialVoltage=0  Measurements=None
  Series RLC Branch1 : spsSeriesRLCBranchLib/Series RLC Branch  Commented=on  LConnTagsString=__new0  RConnTagsString=__new0  BranchType=RL  Resistance=0.0603660020503248  Inductance=0.00288226428630141  SetiL0=off  InitialCurrent=0  Capacitance=1e-6  Setx0=off  InitialVoltage=0  Measurements=None
  Series RLC Branch{4,6..10} (6 alike) : spsSeriesRLCBranchLib/Series RLC Branch  LConnTagsString=__new0  RConnTagsString=__new0  BranchType=RL  Resistance=1.28339880785358  Inductance=0.00408518528456287  SetiL0=off  InitialCurrent=0  Capacitance=1e-6  Setx0=off  InitialVoltage=0  Measurements=None
  Series RLC Branch2 : spsSeriesRLCBranchLib/Series RLC Branch  Commented=on  LConnTagsString=__new0  RConnTagsString=__new0  BranchType=RL  Resistance=0.0402440013668832  Inductance=0.00192150952420094  SetiL0=off  InitialCurrent=0  Capacitance=1e-6  Setx0=off  InitialVoltage=0  Measurements=None
  Series RLC Branch3 : spsSeriesRLCBranchLib/Series RLC Branch  Commented=on  LConnTagsString=__new0  RConnTagsString=__new0  BranchType=RL  Resistance=0.241464008201299  Inductance=0.0115290571452056  SetiL0=off  InitialCurrent=0  Capacitance=1e-6  Setx0=off  InitialVoltage=0  Measurements=None
  Series RLC Branch5 : spsSeriesRLCBranchLib/Series RLC Branch  Commented=on  LConnTagsString=__new0  RConnTagsString=__new0  BranchType=RL  Resistance=0.120732004100650  Inductance=0.00576452857260281  SetiL0=off  InitialCurrent=0  Capacitance=1e-6  Setx0=off  InitialVoltage=0  Measurements=None
  1 : PMIOPort  Side=Left
  Conn2 : PMIOPort  Port=2  Side=Right
  wires:
  Demux/6 -> Ideal Switch5/1
  Demux/5 -> Ideal Switch4/1
  Demux/1 -> Ideal Switch3/1
  Demux/2 -> Ideal Switch/1
  Demux/3 -> Ideal Switch1/1
  Demux/4 -> Ideal Switch2/1
  In1/1 -> Demux/1
  connections:
  Series RLC Branch10/LConn1 -- Ideal Switch5/RConn1
  Series RLC Branch4/LConn1 -- Ideal Switch4/RConn1
  Series RLC Branch9/LConn1 -- Ideal Switch3/RConn1
  Series RLC Branch6/LConn1 -- Ideal Switch2/RConn1
  Series RLC Branch8/LConn1 -- Ideal Switch/RConn1
  Series RLC Branch7/LConn1 -- Ideal Switch1/RConn1
  Series RLC Branch10/RConn1 -- Conn2/RConn1 -- Series RLC Branch8/RConn1 -- Series RLC Branch9/RConn1 -- Series RLC Branch7/RConn1 -- Series RLC Branch6/RConn1 -- Series RLC Branch4/RConn1
  Ideal Switch1/LConn1 -- Ideal Switch2/LConn1 -- Ideal Switch4/LConn1 -- Ideal Switch5/LConn1 -- 1/RConn1 -- Ideal Switch3/LConn1 -- Ideal Switch/LConn1

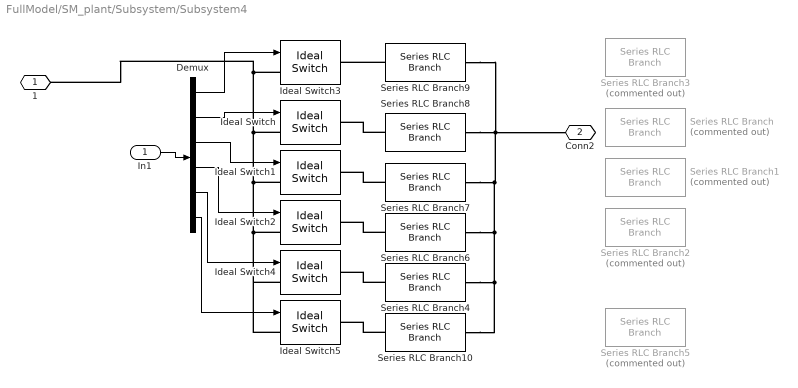
== system FullModel/SM_plant/Subsystem/Subsystem4 ==
  In1 : Inport
  Demux : Demux  Outputs=6
  Ideal Switch{,1..5} (6 alike) : spsIdealSwitchLib/Ideal Switch  Ron=0.001  Lon=0  IC=0  Rs=1e5  Cs=inf  Measurements=off
  Series RLC Branch : spsSeriesRLCBranchLib/Series RLC Branch  Commented=on  LConnTagsString=__new0  RConnTagsString=__new0  BranchType=RL  Resistance=0.241464008201299  Inductance=0.0115290571452056  SetiL0=off  InitialCurrent=0  Capacitance=1e-6  Setx0=off  InitialVoltage=0  Measurements=None
  Series RLC Branch1 : spsSeriesRLCBranchLib/Series RLC Branch  Commented=on  LConnTagsString=__new0  RConnTagsString=__new0  BranchType=RL  Resistance=0.0603660020503248  Inductance=0.00288226428630141  SetiL0=off  InitialCurrent=0  Capacitance=1e-6  Setx0=off  InitialVoltage=0  Measurements=None
  Series RLC Branch{4,6..10} (6 alike) : spsSeriesRLCBranchLib/Series RLC Branch  LConnTagsString=__new0  RConnTagsString=__new0  BranchType=RL  Resistance=1.28339880785358  Inductance=0.00408518528456287  SetiL0=off  InitialCurrent=0  Capacitance=1e-6  Setx0=off  InitialVoltage=0  Measurements=None
  Series RLC Branch2 : spsSeriesRLCBranchLib/Series RLC Branch  Commented=on  LConnTagsString=__new0  RConnTagsString=__new0  BranchType=RL  Resistance=0.0402440013668832  Inductance=0.00192150952420094  SetiL0=off  InitialCurrent=0  Capacitance=1e-6  Setx0=off  InitialVoltage=0  Measurements=None
  Series RLC Branch3 : spsSeriesRLCBranchLib/Series RLC Branch  Commented=on  LConnTagsString=__new0  RConnTagsString=__new0  BranchType=RL  Resistance=0.241464008201299  Inductance=0.0115290571452056  SetiL0=off  InitialCurrent=0  Capacitance=1e-6  Setx0=off  InitialVoltage=0  Measurements=None
  Series RLC Branch5 : spsSeriesRLCBranchLib/Series RLC Branch  Commented=on  LConnTagsString=__new0  RConnTagsString=__new0  BranchType=RL  Resistance=0.120732004100650  Inductance=0.00576452857260281  SetiL0=off  InitialCurrent=0  Capacitance=1e-6  Setx0=off  InitialVoltage=0  Measurements=None
  1 : PMIOPort  Side=Left
  Conn2 : PMIOPort  Port=2  Side=Right
  wires:
  In1/1 -> Demux/1
  Demux/4 -> Ideal Switch2/1
  Demux/3 -> Ideal Switch1/1
  Demux/2 -> Ideal Switch/1
  Demux/1 -> Ideal Switch3/1
  Demux/5 -> Ideal Switch4/1
  Demux/6 -> Ideal Switch5/1
  connections:
  Ideal Switch/LConn1 -- Ideal Switch3/LConn1 -- 1/RConn1 -- Ideal Switch5/LConn1 -- Ideal Switch4/LConn1 -- Ideal Switch2/LConn1 -- Ideal Switch1/LConn1
  Series RLC Branch4/RConn1 -- Series RLC Branch6/RConn1 -- Series RLC Branch7/RConn1 -- Series RLC Branch9/RConn1 -- Series RLC Branch8/RConn1 -- Conn2/RConn1 -- Series RLC Branch10/RConn1
  Series RLC Branch7/LConn1 -- Ideal Switch1/RConn1
  Series RLC Branch8/LConn1 -- Ideal Switch/RConn1
  Series RLC Branch6/LConn1 -- Ideal Switch2/RConn1
  Series RLC Branch9/LConn1 -- Ideal Switch3/RConn1
  Series RLC Branch4/LConn1 -- Ideal Switch4/RConn1
  Series RLC Branch10/LConn1 -- Ideal Switch5/RConn1

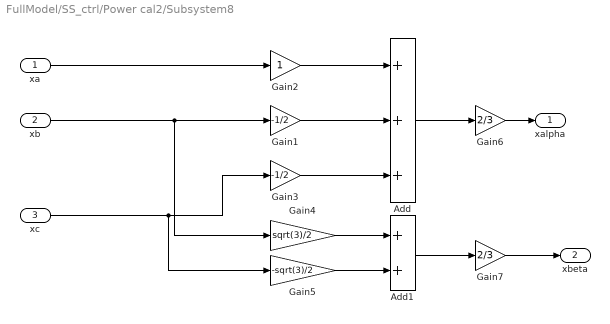
== system FullModel/SS_ctrl/Power cal2/Subsystem8 ==
  xa : Inport
  xb : Inport  Port=2
  xc : Inport  Port=3
  Add : Sum  Inputs=+++
  Add1 : Sum
  Gain1 : Gain  Gain=-1/2
  Gain2 : Gain
  Gain3 : Gain  Gain=-1/2
  Gain4 : Gain  Gain=sqrt(3)/2
  Gain5 : Gain  Gain=-sqrt(3)/2
  Gain6 : Gain  Gain=2/3
  Gain7 : Gain  Gain=2/3
  xalpha : Outport  VectorParamsAs1DForOutWhenUnconnected=off
  xbeta : Outport  Port=2  VectorParamsAs1DForOutWhenUnconnected=off
  wires:
  xc/1 -> Gain5/1, Gain3/1
  Gain6/1 -> xalpha/1
  Add1/1 -> Gain7/1
  Gain3/1 -> Add/3
  Gain1/1 -> Add/2
  xb/1 -> Gain4/1, Gain1/1
  Gain5/1 -> Add1/2
  Gain2/1 -> Add/1
  Add/1 -> Gain6/1
  Gain4/1 -> Add1/1
  Gain7/1 -> xbeta/1
  xa/1 -> Gain2/1

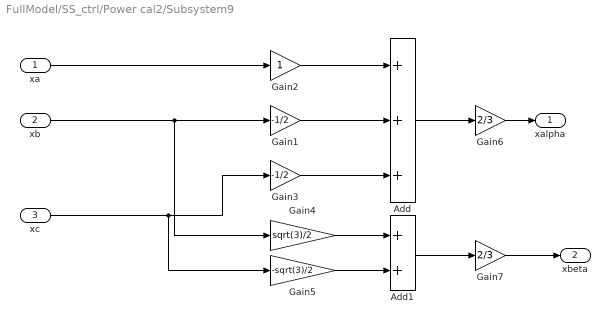
== system FullModel/SS_ctrl/Power cal2/Subsystem9 ==
  xa : Inport
  xb : Inport  Port=2
  xc : Inport  Port=3
  Add : Sum  Inputs=+++
  Add1 : Sum
  Gain1 : Gain  Gain=-1/2
  Gain2 : Gain
  Gain3 : Gain  Gain=-1/2
  Gain4 : Gain  Gain=sqrt(3)/2
  Gain5 : Gain  Gain=-sqrt(3)/2
  Gain6 : Gain  Gain=2/3
  Gain7 : Gain  Gain=2/3
  xalpha : Outport  VectorParamsAs1DForOutWhenUnconnected=off
  xbeta : Outport  Port=2  VectorParamsAs1DForOutWhenUnconnected=off
  wires:
  xa/1 -> Gain2/1
  Gain7/1 -> xbeta/1
  Gain4/1 -> Add1/1
  Add/1 -> Gain6/1
  Gain2/1 -> Add/1
  Gain5/1 -> Add1/2
  xb/1 -> Gain1/1, Gain4/1
  Gain1/1 -> Add/2
  Gain3/1 -> Add/3
  Add1/1 -> Gain7/1
  Gain6/1 -> xalpha/1
  xc/1 -> Gain3/1, Gain5/1

== system FullModel/SS_ctrl/Power cal2/p3 ==
  Alpha : Inport
  Beta : Inport  Port=2
  xalpha : Inport  Port=3
  xbeta : Inport  Port=4
  Add : Sum
  Gain : Gain  Gain=3/2
  Product : Product
  Product1 : Product
  deltay1 : Outport
  wires:
  Product1/1 -> Add/2
  Gain/1 -> deltay1/1
  Product/1 -> Add/1
  Add/1 -> Gain/1
  Alpha/1 -> Product/1
  xalpha/1 -> Product/2
  Beta/1 -> Product1/1
  xbeta/1 -> Product1/2

== system FullModel/SS_ctrl/Power cal2/q3 ==
  Alpha : Inport
  Beta : Inport  Port=2
  xalpha : Inport  Port=3
  xbeta : Inport  Port=4
  Add : Sum  Inputs=+-
  Gain : Gain  Gain=3/2
  Product : Product
  Product1 : Product
  deltay2 : Outport
  wires:
  Add/1 -> Gain/1
  Product/1 -> Add/1
  Gain/1 -> deltay2/1
  Product1/1 -> Add/2
  Beta/1 -> Product/1
  xalpha/1 -> Product/2
  Alpha/1 -> Product1/1
  xbeta/1 -> Product1/2

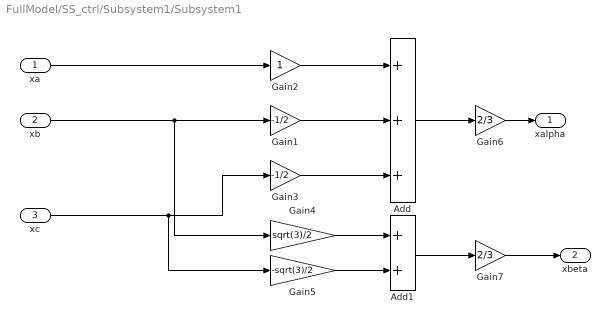
== system FullModel/SS_ctrl/Subsystem1/Subsystem1 ==
  xa : Inport
  xb : Inport  Port=2
  xc : Inport  Port=3
  Add : Sum  Inputs=+++
  Add1 : Sum
  Gain1 : Gain  Gain=-1/2
  Gain2 : Gain
  Gain3 : Gain  Gain=-1/2
  Gain4 : Gain  Gain=sqrt(3)/2
  Gain5 : Gain  Gain=-sqrt(3)/2
  Gain6 : Gain  Gain=2/3
  Gain7 : Gain  Gain=2/3
  xalpha : Outport  VectorParamsAs1DForOutWhenUnconnected=off
  xbeta : Outport  Port=2  VectorParamsAs1DForOutWhenUnconnected=off
  wires:
  xa/1 -> Gain2/1
  Gain7/1 -> xbeta/1
  Gain4/1 -> Add1/1
  Add/1 -> Gain6/1
  Gain2/1 -> Add/1
  Gain5/1 -> Add1/2
  xb/1 -> Gain1/1, Gain4/1
  Gain1/1 -> Add/2
  Gain3/1 -> Add/3
  Add1/1 -> Gain7/1
  Gain6/1 -> xalpha/1
  xc/1 -> Gain3/1, Gain5/1

== system FullModel/SS_ctrl/Subsystem1/Subsystem2 ==
  xalpha : Inport
  xbeta : Inport  Port=2
  wt : Inport  Port=3
  Fcn : Fcn  Expr=cos(u(3))*u(1)+u(2)*sin(u(3))
  Fcn1 : Fcn  Expr=-sin(u(3))*u(1)+u(2)*cos(u(3))
  Mux : Mux  Inputs=3
  xd : Outport  VectorParamsAs1DForOutWhenUnconnected=off
  xq : Outport  Port=2  VectorParamsAs1DForOutWhenUnconnected=off
  wires:
  wt/1 -> Mux/3
  xalpha/1 -> Mux/1
  Fcn1/1 -> xq/1
  xbeta/1 -> Mux/2
  Fcn/1 -> xd/1
  Mux/1 -> Fcn1/1, Fcn/1

== system FullModel/SS_ctrl/Subsystem3/Subsystem1 ==
  xa : Inport
  xb : Inport  Port=2
  xc : Inport  Port=3
  Add : Sum  Inputs=+++
  Add1 : Sum
  Gain1 : Gain  Gain=-1/2
  Gain2 : Gain
  Gain3 : Gain  Gain=-1/2
  Gain4 : Gain  Gain=sqrt(3)/2
  Gain5 : Gain  Gain=-sqrt(3)/2
  Gain6 : Gain  Gain=2/3
  Gain7 : Gain  Gain=2/3
  xalpha : Outport  VectorParamsAs1DForOutWhenUnconnected=off
  xbeta : Outport  Port=2  VectorParamsAs1DForOutWhenUnconnected=off
  wires:
  xc/1 -> Gain5/1, Gain3/1
  Gain6/1 -> xalpha/1
  Add1/1 -> Gain7/1
  Gain3/1 -> Add/3
  Gain1/1 -> Add/2
  xb/1 -> Gain4/1, Gain1/1
  Gain5/1 -> Add1/2
  Gain2/1 -> Add/1
  Add/1 -> Gain6/1
  Gain4/1 -> Add1/1
  Gain7/1 -> xbeta/1
  xa/1 -> Gain2/1

== system FullModel/SS_ctrl/Subsystem3/Subsystem2 ==
  xalpha : Inport
  xbeta : Inport  Port=2
  wt : Inport  Port=3
  Fcn : Fcn  Expr=cos(u(3))*u(1)+u(2)*sin(u(3))
  Fcn1 : Fcn  Expr=-sin(u(3))*u(1)+u(2)*cos(u(3))
  Mux : Mux  Inputs=3
  xd : Outport  VectorParamsAs1DForOutWhenUnconnected=off
  xq : Outport  Port=2  VectorParamsAs1DForOutWhenUnconnected=off
  wires:
  wt/1 -> Mux/3
  Mux/1 -> Fcn/1, Fcn1/1
  Fcn/1 -> xd/1
  xbeta/1 -> Mux/2
  Fcn1/1 -> xq/1
  xalpha/1 -> Mux/1

== system FullModel/SS_ctrl/Subsystem4/Subsystem1 ==
  xa : Inport
  xb : Inport  Port=2
  xc : Inport  Port=3
  Add : Sum  Inputs=+++
  Add1 : Sum
  Gain1 : Gain  Gain=-1/2
  Gain2 : Gain
  Gain3 : Gain  Gain=-1/2
  Gain4 : Gain  Gain=sqrt(3)/2
  Gain5 : Gain  Gain=-sqrt(3)/2
  Gain6 : Gain  Gain=2/3
  Gain7 : Gain  Gain=2/3
  xalpha : Outport  VectorParamsAs1DForOutWhenUnconnected=off
  xbeta : Outport  Port=2  VectorParamsAs1DForOutWhenUnconnected=off
  wires:
  xc/1 -> Gain5/1, Gain3/1
  Gain6/1 -> xalpha/1
  Add1/1 -> Gain7/1
  Gain3/1 -> Add/3
  Gain1/1 -> Add/2
  xb/1 -> Gain4/1, Gain1/1
  Gain5/1 -> Add1/2
  Gain2/1 -> Add/1
  Add/1 -> Gain6/1
  Gain4/1 -> Add1/1
  Gain7/1 -> xbeta/1
  xa/1 -> Gain2/1

== system FullModel/SS_ctrl/Subsystem4/Subsystem2 ==
  xalpha : Inport
  xbeta : Inport  Port=2
  wt : Inport  Port=3
  Fcn : Fcn  Expr=cos(u(3))*u(1)+u(2)*sin(u(3))
  Fcn1 : Fcn  Expr=-sin(u(3))*u(1)+u(2)*cos(u(3))
  Mux : Mux  Inputs=3
  xd : Outport  VectorParamsAs1DForOutWhenUnconnected=off
  xq : Outport  Port=2  VectorParamsAs1DForOutWhenUnconnected=off
  wires:
  Mux/1 -> Fcn/1, Fcn1/1
  Fcn/1 -> xd/1
  xbeta/1 -> Mux/2
  Fcn1/1 -> xq/1
  xalpha/1 -> Mux/1
  wt/1 -> Mux/3

== system FullModel/SS_ctrl/dq-abc/Subsystem2 ==
  xdq : Inport
  wt : Inport  Port=2
  Demux : Demux  Outputs=2
  Fcn2 : Fcn  Expr=u(1)*cos(u(3))-u(2)*sin(u(3))
  Fcn3 : Fcn  Expr=u(1)*sin(u(3))+u(2)*cos(u(3))
  Mux : Mux  Inputs=2
  Mux2 : Mux  Inputs=3
  xalbe : Outport  VectorParamsAs1DForOutWhenUnconnected=off
  wires:
  Mux2/1 -> Fcn2/1, Fcn3/1
  wt/1 -> Mux2/3
  xdq/1 -> Demux/1
  Demux/1 -> Mux2/1
  Demux/2 -> Mux2/2
  Fcn2/1 -> Mux/1
  Fcn3/1 -> Mux/2
  Mux/1 -> xalbe/1

== system FullModel/SS_ctrl/dq-abc/Subsystem3 ==
  xalbe : Inport
  Add : Sum
  Add1 : Sum
  Demux : Demux  Outputs=2
  Gain : Gain
  Gain1 : Gain  Gain=-1/2
  Gain2 : Gain  Gain=sqrt(3)/2
  Gain3 : Gain  Gain=-1/2
  Gain4 : Gain  Gain=-sqrt(3)/2
  Mux : Mux  Inputs=3
  xabc : Outport  VectorParamsAs1DForOutWhenUnconnected=off
  wires:
  Add1/1 -> Mux/3
  Demux/1 -> Gain/1, Gain1/1, Gain3/1
  Gain1/1 -> Add/1
  Add/1 -> Mux/2
  Demux/2 -> Gain2/1, Gain4/1
  Gain3/1 -> Add1/1
  Gain4/1 -> Add1/2
  Gain/1 -> Mux/1
  Gain2/1 -> Add/2
  Mux/1 -> xabc/1
  xalbe/1 -> Demux/1

== matlab function FullModel/SM_plant/Subsystem/MATLAB Function2 ==
  data: t input; s output
function s = RL_switch_logic(t)
%#codegen            % bảo đảm hỗ trợ Code Generation

% Tham số thiết kế
N         = 6;     % số khung R-L
interval  = 20;    % thời gian mỗi khung (giây)

% Xác định khung hiện tại (1…N)
idx = floor(mod(t, N*interval) / interval) + 1;

% Tạo vector điều khiển
s           = zeros(1, N);   % mặc định tất cả switch mở (0)
s(idx)      = 1;             % chỉ khung đang chọn đóng (1)
end
